simulink model "Lecture7_Model2"  (R2021a)
settings: Solver=VariableStepAuto  StartTime=0  StopTime=inf  MaxStep=1e-5  RelTol=1e-3
InitFcn:
  | Init_File_7
undefined symbols (not defined in the file): Bulb_R, C, Encoder_Gain, Generator_Voltage_Gain, P1, P2, R, Torque_Constant
libraries: fl_lib x13, nesl_utility x8, simulink x2, sdl_lib x1
settings Model: Creator=Admin  LastModifiedBy=Admin
settings SolverCC: InitialStep=1e-5

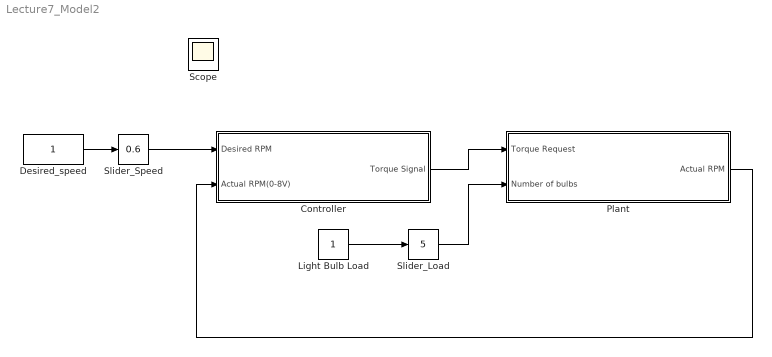
== system Lecture7_Model2 ==
  "Controller " : Subsystem
  Desired_speed : Constant
  Light Bulb Load : Constant
  Plant : Subsystem
  Slider_Load : simulink/Math Operations/Slider Gain  gain=5  low=0  high=6
  Slider_Speed : simulink/Math Operations/Slider Gain  gain=0.6  low=0  high=1
  Scope : Scope
  wires:
  "Controller "/1(Torque Signal) -> Plant/1(Torque Request)
  Desired_speed/1 -> Slider_Speed/1
  Plant/1(Actual RPM) -> "Controller "/2(Actual RPM(0-8V))
  Slider_Speed/1 -> "Controller "/1(Desired RPM)
  Light Bulb Load/1 -> Slider_Load/1
  Slider_Load/1 -> Plant/2(Number of bulbs)

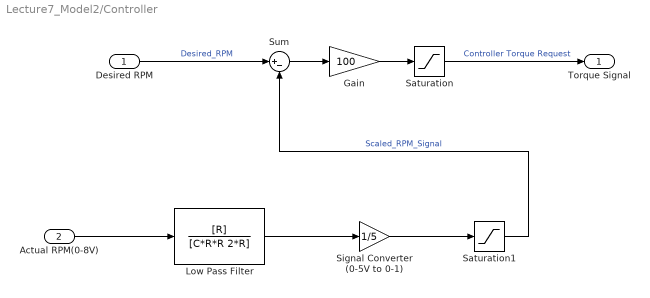
== system Lecture7_Model2/Controller  ==
  Desired RPM : Inport
  Actual RPM(0-8V) : Inport  Port=2
  Gain : Gain  Gain=100
  Low Pass Filter : TransferFcn  Numerator=[R]  Denominator=[C*R*R 2*R]
  Saturation : Saturate  UpperLimit=1  LowerLimit=0
  Saturation1 : Saturate  UpperLimit=1  LowerLimit=0
  Signal Converter (0-5V to 0-1) : Gain  Gain=1/5
  Sum : Sum  Inputs=|+-
  Torque Signal : Outport
  wires:
  Desired RPM/1 -> Sum/1  "Desired_RPM"
  Sum/1 -> Gain/1
  Gain/1 -> Saturation/1
  Saturation/1 -> Torque Signal/1  "Controller Torque Request"
  Actual RPM(0-8V)/1 -> Low Pass Filter/1
  Low Pass Filter/1 -> Signal Converter (0-5V to 0-1)/1
  Signal Converter (0-5V to 0-1)/1 -> Saturation1/1
  Saturation1/1 -> Sum/2  "Scaled_RPM_Signal"

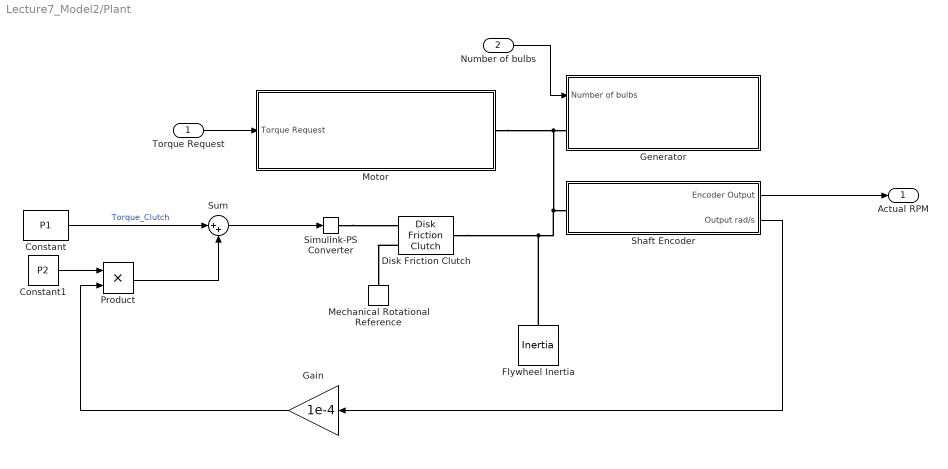
== system Lecture7_Model2/Plant ==
  Torque Request : Inport
  Number of bulbs : Inport  Port=2
  Constant : Constant  Value=P1
  Constant1 : Constant  Value=P2
  Disk Friction Clutch : sdl_lib/Clutches/Disk Friction Clutch  geometry_model=sdl.enum.friction_geometry.radius  r_eff=1 m  d_o=150 mm  d_i=100 mm  nS=1  piston_area=1 m^2  unidirectional=sdl.enum.directionality.unidirectional  friction_model=sdl.enum.friction_model_TLU_thermal.fixed  mu_w_vector=[0, 100, 1000] rad/s  temperature_TLU=[280, 300, 320] K  mu_static=1  mu_static_vector=[.4, .38, .36]  mu_coulomb=1  mu_coulomb_vector=[.3, .22, .19]  mu_coulomb_temp_vector=[.3, .28, .25]  mu_coulomb_matrix=[.34, .32, .3; .3, .28, .25; .25, .2, .15]  mu_interp_method=simscape.enum.interpolation.linear  mu_extrap_method=simscape.enum.extrapolation.linear  d_f=1  w_tol=0.001 rad/s  pressure_min=0 Pa  mu_visc=0 N*m/(rad/s)  initial_state_locked=sdl.enum.initial_lock.unlocked  enable_faults=simscape.enum.onoff.off  fault_type=sdl.enum.clutchFault.lock  external_fault=simscape.enum.onoff.off  temporal_fault=simscape.enum.onoff.off  fault_time=5 s  report_fault=simscape.enum.assert.action.none  thermal_mass=50 kJ/K  T_init=300 K
      settings: SourceProductBaseCode=LD  InternalSimscapePortConfiguration="{\"Bottom\":[],\"Left\":[{\"id\":\"P\",\"label\":\"P\",\"type\":\"input\"},{\"id\":\"B\",\"label\":\"B\",\"type\":\"foundation.mechanical.rotational.rotational\"}],\"Right\":[{\"id\":\"F\",\"label\":\"F\",\"type\":\"foundation.mechanical.rotational.rotational\"}],\"Top\":[]}"
  Flywheel Inertia : fl_lib/Mechanical/Rotational Elements/Inertia  inertia=Flywheel_Inertia kg*m^2  num_ports=foundation.enum.numPorts2.one  w_specify=off  w_priority=High  w=0 rad/s  w_nominal_specify=off  w_nominal_unit=rad/s  w_nominal_value=1  t_specify=off  t_priority=None  t=0 N*m  t_nominal_specify=off  t_nominal_unit=N*m  t_nominal_value=1
  Gain : Gain  Gain=1e-4
  "Generator " : Subsystem
  Mechanical Rotational Reference : fl_lib/Mechanical/Rotational Elements/Mechanical Rotational Reference
  "Motor " : Subsystem
  Product : Product
  Shaft Encoder : Subsystem
  Simulink-PS Converter : nesl_utility/Simulink-PS Converter  PhysicalDomain=network_engine_domain  SubClassName=ps_input  LeftPortType=input  RightPortType=output  PseudoPeriodic=off  Frequencies=[]  NoiseDistribution=none  NoiseParameters=[]  Unit=1  AffineConversion=off  FilteringAndDerivatives=provide  SimscapeFilterOrder=1  InputFilterTimeConstant=0.001  UdotUserProvided=0
      settings: SourceProductBaseCode=PW,SS
  Sum : Sum  Inputs=|++
  Actual RPM : Outport
  wires:
  Torque Request/1 -> "Motor "/1(Torque Request)
  Shaft Encoder/1(Encoder Output) -> Actual RPM/1
  Number of bulbs/1 -> "Generator "/1(Number of bulbs)
  Constant/1 -> Sum/1  "Torque_Clutch"
  Sum/1 -> Simulink-PS Converter/1
  Constant1/1 -> Product/1
  Shaft Encoder/2(Output rad/s) -> Gain/1
  Gain/1 -> Product/2
  Product/1 -> Sum/2
  connections:
  "Motor "/RConn1 -- Disk Friction Clutch/RConn1 -- Flywheel Inertia/LConn1 -- Shaft Encoder/LConn1 -- "Generator "/LConn1
  Disk Friction Clutch/LConn2 -- Mechanical Rotational Reference/LConn1
  Simulink-PS Converter/RConn1 -- Disk Friction Clutch/LConn1

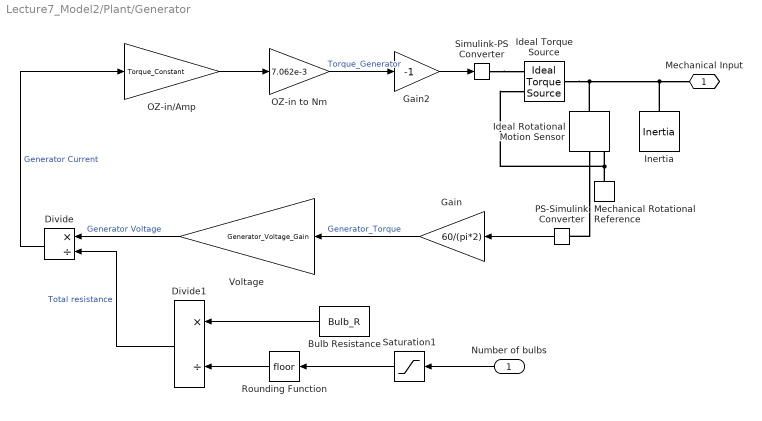
== system Lecture7_Model2/Plant/Generator  ==
  Number of bulbs : Inport
  Bulb Resistance : Constant  Value=Bulb_R
  Divide : Product  Inputs=*/
  Divide1 : Product  Inputs=*/
  Gain : Gain  Gain=60/(pi*2)
  Gain2 : Gain  Gain=-1
  Ideal Rotational Motion Sensor : fl_lib/Mechanical/Mechanical Sensors/Ideal Rotational Motion Sensor  wrap_angle=simscape.enum.onoff.off  offset=0 rad
  Ideal Torque Source : fl_lib/Mechanical/Mechanical Sources/Ideal Torque Source
  Inertia : fl_lib/Mechanical/Rotational Elements/Inertia  inertia=Generator_Inertia kg*m^2  num_ports=foundation.enum.numPorts2.one  w_specify=on  w_priority=High  w=0 rpm  w_nominal_specify=off  w_nominal_unit=rad/s  w_nominal_value=1  t_specify=off  t_priority=None  t=0 N*m  t_nominal_specify=off  t_nominal_unit=N*m  t_nominal_value=1
  Mechanical Rotational Reference : fl_lib/Mechanical/Rotational Elements/Mechanical Rotational Reference
  OZ-in to Nm : Gain  Gain=7.062e-3
  OZ-in/Amp : Gain  Gain=Torque_Constant
  PS-Simulink Converter : nesl_utility/PS-Simulink Converter  PhysicalDomain=network_engine_domain  SubClassName=ps_output  LeftPortType=input  RightPortType=output  PseudoPeriodic=off  Frequencies=[]  Unit=inherit  AffineConversion=off
      settings: SourceProductBaseCode=PW,SS
  Rounding Function : Rounding
  Saturation1 : Saturate  UpperLimit=6  LowerLimit=0
  Simulink-PS Converter : nesl_utility/Simulink-PS Converter  PhysicalDomain=network_engine_domain  SubClassName=ps_input  LeftPortType=input  RightPortType=output  PseudoPeriodic=off  Frequencies=[]  NoiseDistribution=none  NoiseParameters=[]  Unit=1  AffineConversion=off  FilteringAndDerivatives=filter  SimscapeFilterOrder=1  InputFilterTimeConstant=0.001  UdotUserProvided=0
      settings: SourceProductBaseCode=PW,SS
  Voltage : Gain  Gain=Generator_Voltage_Gain
  Mechanical Input : PMIOPort  Side=Left
  wires:
  PS-Simulink Converter/1 -> Gain/1
  Gain2/1 -> Simulink-PS Converter/1
  Number of bulbs/1 -> Saturation1/1
  Saturation1/1 -> Rounding Function/1
  Rounding Function/1 -> Divide1/2
  Bulb Resistance/1 -> Divide1/1
  Gain/1 -> Voltage/1  "Generator_Torque"
  Divide1/1 -> Divide/2  "Total resistance"
  Voltage/1 -> Divide/1  "Generator Voltage"
  OZ-in/Amp/1 -> OZ-in to Nm/1
  OZ-in to Nm/1 -> Gain2/1  "Torque_Generator"
  Divide/1 -> OZ-in/Amp/1  "Generator Current"
  connections:
  Ideal Torque Source/LConn1 -- Inertia/LConn1 -- Mechanical Input/RConn1 -- Ideal Rotational Motion Sensor/LConn1
  Simulink-PS Converter/RConn1 -- Ideal Torque Source/RConn1
  Ideal Rotational Motion Sensor/RConn2 -- PS-Simulink Converter/LConn1
  Mechanical Rotational Reference/LConn1 -- Ideal Torque Source/RConn2 -- Ideal Rotational Motion Sensor/RConn1

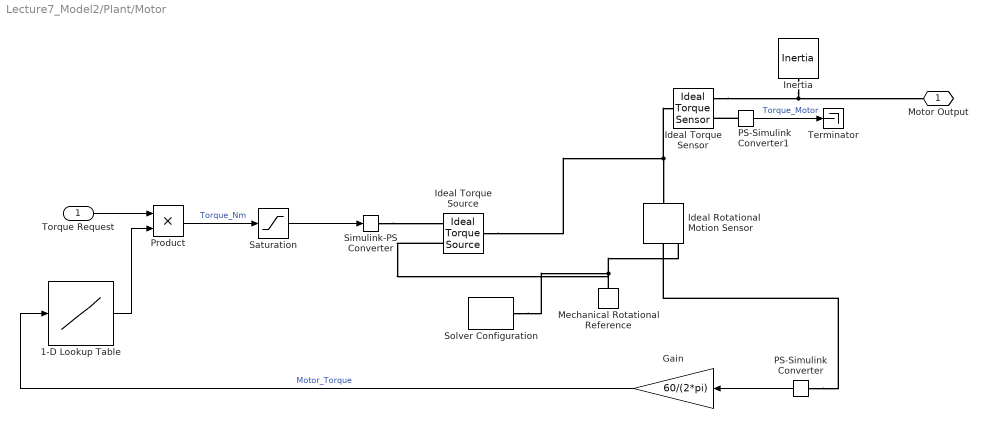
== system Lecture7_Model2/Plant/Motor  ==
  Torque Request : Inport
  1-D Lookup Table : Lookup_n-D  NumberOfTableDimensions=1  BreakpointsForDimension1=[0 1000 2000 3000 4000]  Table=[0.4 0.4 0.3 0.2 0]  InternalRulePriority=Speed  RndMeth=Simplest  InputSameDT=on
  Gain : Gain  Gain=60/(2*pi)
  Ideal Rotational Motion Sensor : fl_lib/Mechanical/Mechanical Sensors/Ideal Rotational Motion Sensor  wrap_angle=simscape.enum.onoff.off  offset=0 deg
  Ideal Torque Sensor : fl_lib/Mechanical/Mechanical Sensors/Ideal Torque Sensor
  Ideal Torque Source : fl_lib/Mechanical/Mechanical Sources/Ideal Torque Source
  Inertia : fl_lib/Mechanical/Rotational Elements/Inertia  inertia=Motor_Inertia kg*m^2  num_ports=foundation.enum.numPorts2.one  w_specify=on  w_priority=High  w=0 rpm  w_nominal_specify=off  w_nominal_unit=rad/s  w_nominal_value=1  t_specify=off  t_priority=None  t=0 N*m  t_nominal_specify=off  t_nominal_unit=N*m  t_nominal_value=1
  Mechanical Rotational Reference : fl_lib/Mechanical/Rotational Elements/Mechanical Rotational Reference
  PS-Simulink Converter : nesl_utility/PS-Simulink Converter  PhysicalDomain=network_engine_domain  SubClassName=ps_output  LeftPortType=input  RightPortType=output  PseudoPeriodic=off  Frequencies=[]  Unit=inherit  AffineConversion=off
      settings: SourceProductBaseCode=PW,SS
  PS-Simulink Converter1 : nesl_utility/PS-Simulink Converter  PhysicalDomain=network_engine_domain  SubClassName=ps_output  LeftPortType=input  RightPortType=output  PseudoPeriodic=off  Frequencies=[]  Unit=inherit  AffineConversion=off
      settings: SourceProductBaseCode=PW,SS
  Product : Product
  Saturation : Saturate  UpperLimit=inf  LowerLimit=0
  Simulink-PS Converter : nesl_utility/Simulink-PS Converter  PhysicalDomain=network_engine_domain  SubClassName=ps_input  LeftPortType=input  RightPortType=output  PseudoPeriodic=off  Frequencies=[]  NoiseDistribution=none  NoiseParameters=[]  Unit=1  AffineConversion=off  FilteringAndDerivatives=filter  SimscapeFilterOrder=1  InputFilterTimeConstant=0.001  UdotUserProvided=0
      settings: SourceProductBaseCode=PW,SS
  Solver Configuration : nesl_utility/Solver Configuration  PhysicalDomain=network_engine_domain  SubClassName=solver  LeftPortType=input  RightPortType=generic  Tones=[]  Harmonics=[]  SimulateNoise=off  Profile=off  UseLocalSampling=off  EnableSwitchedLinearOptims=on  FrequencyDomain=off  UseCCode=off  RelTol=0.001  AbsTol=1e-06  MinStep=1e-09  ToWorkspace=off  RevertToSquareIcSolve=off  NumHomotopyIterations=100  PhasorMode=off  PhasorModeNumHarmonics=1  DoDC=off  ResidualTolerance=1e-09  UseLocalSolver=off  LocalSolverChoice=NE_BACKWARD_EULER_ADVANCER  LocalSolverSampleTime=0.001  DoFixedCost=off  MaxNonlinIter=3  MaxModeIter=2  ComputeImpulses=off  ImpulseIterations=2  LinearAlgebra=auto  EquationFormulation=NE_TIME_EF  DelaysMemoryBudget=1024  AutomaticFiltering=on  FilteringTimeConstant=0.001  PartitionStorageMethod=AS_NEEDED  PartitionMemoryBudget=1024  PartitionMethod=ROBUST
      settings: SourceProductBaseCode=PW,SS
  Terminator : Terminator
  Motor Output : PMIOPort  Side=Right
  wires:
  PS-Simulink Converter/1 -> Gain/1
  1-D Lookup Table/1 -> Product/2
  Torque Request/1 -> Product/1
  Gain/1 -> 1-D Lookup Table/1  "Motor_Torque"
  Product/1 -> Saturation/1  "Torque_Nm"
  Saturation/1 -> Simulink-PS Converter/1
  PS-Simulink Converter1/1 -> Terminator/1  "Torque_Motor"
  connections:
  Ideal Torque Sensor/RConn1 -- Inertia/LConn1 -- Motor Output/RConn1
  Mechanical Rotational Reference/LConn1 -- Solver Configuration/RConn1 -- Ideal Torque Source/RConn2 -- Ideal Rotational Motion Sensor/RConn1
  Simulink-PS Converter/RConn1 -- Ideal Torque Source/RConn1
  PS-Simulink Converter/LConn1 -- Ideal Rotational Motion Sensor/RConn2
  Ideal Torque Source/LConn1 -- Ideal Torque Sensor/LConn1 -- Ideal Rotational Motion Sensor/LConn1
  PS-Simulink Converter1/LConn1 -- Ideal Torque Sensor/RConn2

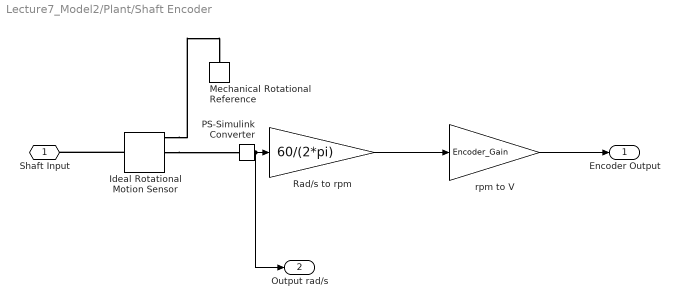
== system Lecture7_Model2/Plant/Shaft Encoder ==
  Ideal Rotational Motion Sensor : fl_lib/Mechanical/Mechanical Sensors/Ideal Rotational Motion Sensor  wrap_angle=simscape.enum.onoff.off  offset=0 rad
  Mechanical Rotational Reference : fl_lib/Mechanical/Rotational Elements/Mechanical Rotational Reference
  PS-Simulink Converter : nesl_utility/PS-Simulink Converter  PhysicalDomain=network_engine_domain  SubClassName=ps_output  LeftPortType=input  RightPortType=output  PseudoPeriodic=off  Frequencies=[]  Unit=inherit  AffineConversion=off
      settings: SourceProductBaseCode=PW,SS
  Rad/s to rpm : Gain  Gain=60/(2*pi)
  rpm to V : Gain  Gain=Encoder_Gain
  Shaft Input : PMIOPort  Side=Left
  Encoder Output : Outport
  Output rad/s : Outport  Port=2
  wires:
  PS-Simulink Converter/1 -> Output rad/s/1, Rad/s to rpm/1
  Rad/s to rpm/1 -> rpm to V/1
  rpm to V/1 -> Encoder Output/1
  connections:
  Ideal Rotational Motion Sensor/LConn1 -- Shaft Input/RConn1
  Ideal Rotational Motion Sensor/RConn1 -- Mechanical Rotational Reference/LConn1
  Ideal Rotational Motion Sensor/RConn2 -- PS-Simulink Converter/LConn1
